simulink model "Self_Excited_Induction_Generator_SEIG"  (R2025a)
settings: Solver=ode23tb  StartTime=0.0  StopTime=10.0  MaxStep=1e-4  RelTol=1e-3
libraries: spsThreePhaseSeriesRLCBranchLib x2, spsGroundLib x2, spsDCVoltageSourceLib x2, spsAsynchronousMachineSIUnitsLib x1, spsDCMachineLib x1, spsRMSLib x1, spsVoltageMeasurementLib x1, sps_lib x1
settings Model: Creator=Jawad  LastModifiedBy=Jawad

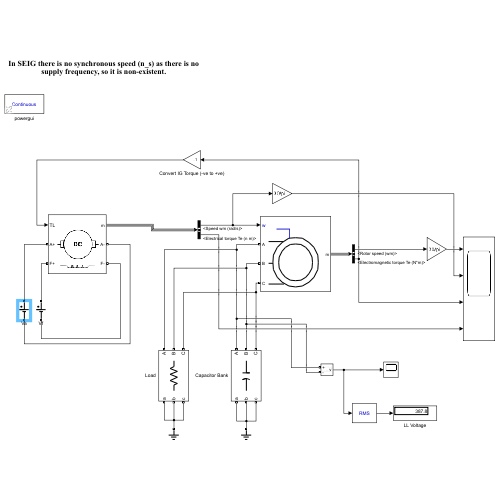
[thumbnail: Simulink's stored preview of the top-level diagram]
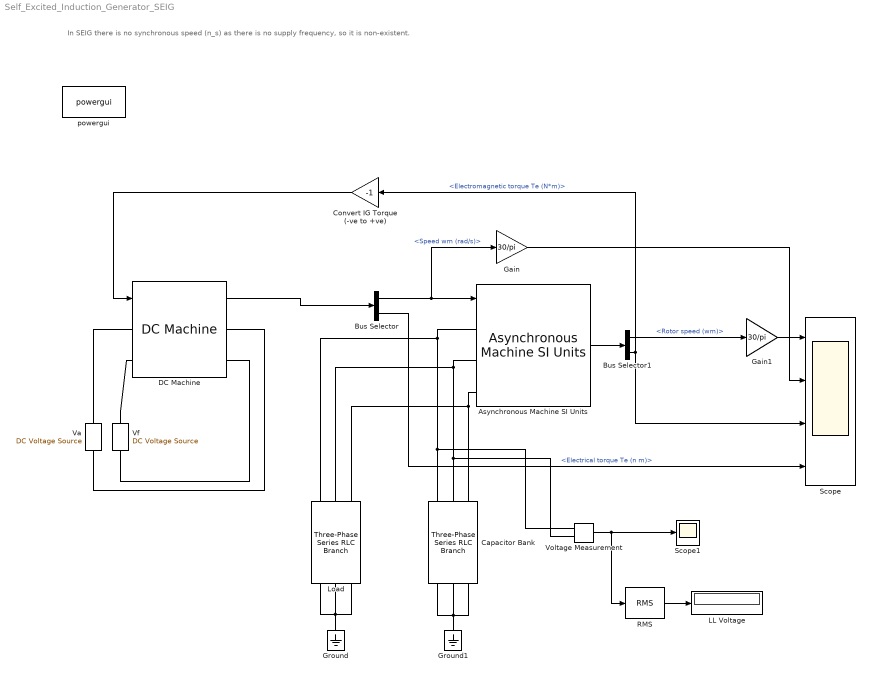
== system Self_Excited_Induction_Generator_SEIG ==
  note: In SEIG there is no synchronous speed (n_s) as there is no supply frequency, so it is non-existent.
  Asynchronous Machine SI Units : spsAsynchronousMachineSIUnitsLib/Asynchronous Machine SI Units  RotorType=Squirrel-cage  PresetModel="15:  5.4 HP (4KW)   400 V  50Hz 1430 RPM"  MechanicalLoad=Speed w  ShowDetailedParameters=on  ReferenceFrame=Stationary  Units=SI  MeasurementBus=off  NominalParameters=[4000 400 50]  VoltageRatio=1  Stator=[1.405 0.005839]  Rotor=[1.395 0.005839]  Cage1=[0.4155 0.002066]  Cage2=[0.4168 0.0003495]  Lm=0.1722  Mechanical=[0.0131 0.002985 2]  PolePairs=2  InitialConditions=[1 0 1 1 1 0 -120 120]  SimulateSaturation=off  Saturation=[14.03593122, 27.81365428, 53.79336849, 72.68890987, 97.98006896, 148.6815601, 215.7428561, 302.9841135, 428.7778367 ; 230, 322, 414, 460, 506, 552, 598, 644, 690]  LoadFlowParameters=1492000  TsPowergui=0  TsBlock=-1  IterativeModel=Trapezoidal non iterative  IterativeDiscreteModel=Trapezoidal non iterative  Pmec=1.492e+006
  Bus Selector : BusSelector  OutputSignals=Speed wm (rad/s),Electrical torque Te (n m)
  Bus Selector1 : BusSelector  OutputSignals=Mechanical.Rotor speed (wm),Mechanical.Electromagnetic torque Te (N*m)
  Capacitor Bank : spsThreePhaseSeriesRLCBranchLib/Three-Phase Series RLC Branch  LConnTagsString=A|B|C  RConnTagsString=A|B|C  BranchType=C  Resistance=1  Inductance=1e-3  Capacitance=53e-6  Measurements=None
  Convert IG Torque (-ve to +ve) : Gain  Gain=-1
  DC Machine : spsDCMachineLib/DC Machine  PresetModel=01: 5HP 240V 1750RPM Field:300V  MechanicalLoad=Torque TL  FieldType=Wound  ShowDetailedParameters=on  MeasurementBus=off  RLa=[2.581 0.028]  RLf=[281.2 156]  Laf=0.9483  MachineConstant=Torque constant (N.m/A)  Ke=1.8  Kt=1.8  J=0.02215  Bm=0.002953  Tf=0.5161  w0=1  Ifinit=1.06685633001422  TsPowergui=0  TsBlock=-1
  Gain : Gain  Gain=30/pi
  Gain1 : Gain  Gain=30/pi
  Ground : spsGroundLib/Ground  LConnTagsString=a
  Ground1 : spsGroundLib/Ground  LConnTagsString=a
  LL Voltage : Display
  Load : spsThreePhaseSeriesRLCBranchLib/Three-Phase Series RLC Branch  LConnTagsString=A|B|C  RConnTagsString=A|B|C  BranchType=R  Resistance=50  Inductance=1e-3  Capacitance=1e-6  Measurements=None
  RMS : spsRMSLib/RMS  TrueRMS=off  Freq=50  RMSInit=0  Ts=0
  Scope : Scope  NumInputPorts=4
      settings: ActiveDisplayYMinimum=-268.27129546540812  ActiveDisplayYMaximum=2509.9346250438111
  Scope1 : Scope
      settings: ActiveDisplayYMinimum=-24.519008816378808  ActiveDisplayYMaximum=11.830015485295279
  Va : spsDCVoltageSourceLib/DC Voltage Source  Amplitude=240  Measurements=None
  Vf : spsDCVoltageSourceLib/DC Voltage Source  Amplitude=300  Measurements=None
  Voltage Measurement : spsVoltageMeasurementLib/Voltage Measurement  PhasorSimulation=off  OutputType=Complex  PSBequivalent=0
  powergui : sps_lib/powergui  Priority=1  SimulationMode=Continuous  SampleTime=50e-6  frequency=60  Iterations=50  frequencyindice=50  Pbase=100e6  ErrMax=1e-4  UnitsV=kV  UnitsW=MW  buscounter=0  FunctionMessages=off  echomessages=off  EnableUseOfTLC=off  CurrentSourceSwitches=off  DisableSnubberDevices=off  DisableRonSwitches=off  DisableVfSwitches=off  DisplayEquations=off  AutomaticDiscreteSolvers=off  SolverType=Tustin/Backward Euler (TBE)  Interpol=off  ExternalGateDelay=off  methode=off  Ts=100  x0status=blocks  SPID=on  SwTol=0  HookPort=off  NonlinearTolerance=1e-4  nMaxIteration=100  ContinueOnMaxIteration=off  RestoreLinks=warning  ResistiveCurrentMeasurement=off  Frange=[0:2:500]  Ylog=off  Xlog=on  ShowGrid=off  save=off  variable=ZData  structure=0  ZoomFFT=off  StartTime=0.0  cycles=1  DisplayStyle=1  fundamental=60  FreqAxis=off  MaxFrequency=1000  frequencyindicesteady=1  RmsSteady=1  display=off
  wires:
  DC Machine/1 -> Bus Selector/1
  Bus Selector/1 -> Gain/1, Asynchronous Machine SI Units/1  "<Speed wm (rad/s)>"
  Asynchronous Machine SI Units/1 -> Bus Selector1/1
  Bus Selector1/2 -> Scope/3, Convert IG Torque (-ve to +ve)/1  "<Electromagnetic torque Te (N*m)>"
  Convert IG Torque (-ve to +ve)/1 -> DC Machine/1
  Bus Selector1/1 -> Gain1/1  "<Rotor speed (wm)>"
  Gain/1 -> Scope/2
  Bus Selector/2 -> Scope/4  "<Electrical torque Te (n m)>"
  Voltage Measurement/1 -> RMS/1, Scope1/1
  RMS/1 -> LL Voltage/1
  Gain1/1 -> Scope/1
  connections:
  Va/RConn1 -- DC Machine/LConn1
  Va/LConn1 -- DC Machine/RConn1
  Vf/RConn1 -- DC Machine/LConn2
  Vf/LConn1 -- DC Machine/RConn2
  Capacitor Bank/RConn1 -- Capacitor Bank/RConn2 -- Ground1/LConn1 -- Capacitor Bank/RConn3
  Capacitor Bank/LConn3 -- Load/LConn3 -- Asynchronous Machine SI Units/LConn3
  Capacitor Bank/LConn2 -- Voltage Measurement/LConn2 -- Load/LConn2 -- Asynchronous Machine SI Units/LConn2
  Capacitor Bank/LConn1 -- Voltage Measurement/LConn1 -- Load/LConn1 -- Asynchronous Machine SI Units/LConn1
  Load/RConn1 -- Load/RConn2 -- Ground/LConn1 -- Load/RConn3
